simulink model "PosControl_Sim_RPT"  (R2023b)
settings: Solver=ode4  StartTime=0.0  StopTime=3.35  FixedStep=0.001  RelTol=1e-3
InitFcn:
  | Init_control;
values from neighbouring files (symbols this model uses):
  CONSTANTS_ONE_G = 9.8    [Init_control.m]
  DEG2RAD = 0.0174533    [Init_control.m]
  F_xy = [(wn^2+2*sigma*wn*ki)/eps^2, (2*sigma*wn+ki)/eps, ki*wn^2/eps^3, -(wn^2+2*sigma*wn*ki)/eps^2, -(2*sigma*wn+ki)/eps]    [Init_control.m]
  F_z = [(wn^2+2*sigma*wn*ki)/eps^2, (2*sigma*wn+ki)/eps, ki*wn^2/eps^3, -(wn^2+2*sigma*wn*ki)/eps^2, -(2*sigma*wn+ki)/eps]    [Init_control.m]
  FLT_EPSILON = 1e-5    (= 1e-05)    [Init_control.m]
  MAX_CONTROL_ANGLE_RATE_PITCH = 220    [Init_control.m]
  MAX_CONTROL_ANGLE_RATE_ROLL = 220    [Init_control.m]
  MAX_CONTROL_ANGLE_RATE_Y = 200    [Init_control.m]
  MAX_CONTROL_VELOCITY_XY = 5*2    (= 10)    [Init_control.m]
  MAX_CONTROL_VELOCITY_Z = 3*2    (= 6)    [Init_control.m]
  MC_PITCH_P = 6.5    [Init_control.m]
  MC_PITCHRATE_D = 0.0005    [Init_control.m]
  MC_PITCHRATE_I = 0.2    [Init_control.m]
  MC_PITCHRATE_P = 0.06    [Init_control.m]
  MC_ROLL_P = 11.5    [Init_control.m]
  MC_ROLLRATE_D = 0.0005    [Init_control.m]
  MC_ROLLRATE_I = 0.2    [Init_control.m]
  MC_ROLLRATE_P = 0.055    [Init_control.m]
  MC_YAW_P = 2.8    [Init_control.m]
  MC_YAW_WEIGHT = 0.4    [Init_control.m]
  MC_YAWRATE_D = 0.00    (= 0)    [Init_control.m]
  MC_YAWRATE_I = 0.1    [Init_control.m]
  MC_YAWRATE_P = 0.2    [Init_control.m]
  MPC_THR_MAX = 0.9    [Init_control.m]
  MPC_THR_MIN = 0.06    [Init_control.m]
  MPC_THR_XY_MARG = 0.3    [Init_control.m]
  MPC_TILTMAX_AIR = 90    [Init_control.m]
  Saturation_I_az = 5    [Init_control.m]
  Saturation_I_RP_Max = 0.3    [Init_control.m]
  Saturation_I_RP_Min = -0.3    [Init_control.m]
  Saturation_I_Y_Max = 0.2    [Init_control.m]
  Saturation_I_Y_Min = -0.2    [Init_control.m]
  THR_HOVER = 0.331    [Init_control.m]
undefined symbols (not defined in the file or in its folder): DiscIntNeverNeededParam, earthRadius, ModelInit_AngEuler, ModelInit_PosE, ModelInit_Rads, ModelInit_RateB, ModelInit_VelB, ModelParam_envGravityAcc, ModelParam_motorCp, ModelParam_motorCr, ModelParam_motorJm, ModelParam_motorT, ModelParam_motorWb, ModelParam_rotorCm, ModelParam_rotorCt, ModelParam_uavCCm, ModelParam_uavCd, ModelParam_uavJ, ModelParam_uavMass, ModelParam_uavR
libraries: simulink x4, sharedutil x2, aerolibfltsims x2, aerolibanimutils x1
(part 2 of 2)

== matlab function PosControl_Sim_RPT/Control System/Control System/position_control/MATLAB Function1 ==
  data: accx_sp input; thr_sp output; accy_sp input; accz_sp input; CONSTANTS_ONE_G input; DEG2RAD input; MPC_TILTMAX_AIR input; THR_HOVER input; MPC_THR_MIN input; FLT_EPSILON input
function thr_sp = accelerationControl(accx_sp, accy_sp, accz_sp, CONSTANTS_ONE_G, DEG2RAD, MPC_TILTMAX_AIR, THR_HOVER, MPC_THR_MIN, FLT_EPSILON)

selMethod = 2;

if selMethod == 1 % this original method implmented in PX4

    lim_thr_min = MPC_THR_MIN; 

    acc_sp = [accx_sp, accy_sp, accz_sp]';
    thr_sp = zeros(3,1);

    % Assume standard acceleration due to gravity in vertical direction for attitude generation
    body_z = [-acc_sp(1), -acc_sp(2), CONSTANTS_ONE_G]';
    body_z = body_z / norm(body_z);

    lim_tilt = MPC_TILTMAX_AIR * DEG2RAD; 
    limitTilt(body_z, [0, 0, 1]', lim_tilt, FLT_EPSILON);

    % Scale thrust assuming hover thrust produces standard gravity
    hover_thrust = THR_HOVER; 
    collective_thrust = acc_sp(3) * (hover_thrust / CONSTANTS_ONE_G) - hover_thrust;

    % Project thrust to planned body attitude
    collective_thrust = collective_thrust / dot( [0, 0, 1]', body_z );

    collective_thrust = min(collective_thrust, -lim_thr_min);
    thr_sp = body_z * collective_thrust;

else
    lim_thr_min = MPC_THR_MIN; 

    acc_sp = [accx_sp, accy_sp, accz_sp]';
    thr_sp = zeros(3,1);

    % Assume standard acceleration due to gravity in vertical direction for attitude generation
    % body_z = [-acc_sp(1), -acc_sp(2), CONSTANTS_ONE_G]';
    if acc_sp(3) < CONSTANTS_ONE_G 
        body_z = [-acc_sp(1), -acc_sp(2), -acc_sp(3) + CONSTANTS_ONE_G]';
    else
        body_z = [-acc_sp(1), -acc_sp(2), 0]'; % Prevent the drone from flipping upside down
        acc_sp(3) = CONSTANTS_ONE_G; % ma
    end
    body_z = body_z / norm(body_z);

    lim_tilt = MPC_TILTMAX_AIR * DEG2RAD; 
    limitTilt(body_z, [0, 0, 1]', lim_tilt, FLT_EPSILON);

    % Scale thrust assuming hover thrust produces standard gravity
    hover_thrust = THR_HOVER; 
    % collective_thrust = acc_sp(3) * (hover_thrust / CONSTANTS_ONE_G) - hover_thrust;
    
    collective_thrust = - norm(acc_sp + [0, 0, -CONSTANTS_ONE_G]') * (hover_thrust / CONSTANTS_ONE_G); 

    % Project thrust to planned body attitude
%     if dot( [0, 0, 1]', body_z ) > FLT_EPSILON
%         collective_thrust = collective_thrust / dot( [0, 0, 1]', body_z );
%     else
%         collective_thrust = norm(acc_sp) * (hover_thrust / CONSTANTS_ONE_G) - hover_thrust;
%     end

    collective_thrust = min(collective_thrust, -lim_thr_min);
    thr_sp = body_z * collective_thrust;
end 

end


function body_unit = limitTilt(body_unit, world_unit, max_angle, FLT_EPSILON )
    
    % determine tilt
	dot_product_unit = dot(body_unit, world_unit);
	angle = acos(dot_product_unit);
	
    % limit tilt
	angle = min(angle, max_angle);
	rejection = body_unit - (dot_product_unit * world_unit);

	% corner case exactly parallel vectors
	if  norm(rejection)^2 < FLT_EPSILON  
		rejection(1) = 1.0;
    end

	body_unit = cos(angle) * world_unit + sin(angle) * ( rejection/norm(rejection) );

end


% void limitTilt(Vector3f &body_unit, const Vector3f &world_unit, const float max_angle)
% {
% 	// determine tilt
% 	const float dot_product_unit = body_unit.dot(world_unit);
% 	float angle = acosf(dot_product_unit);
% 	// limit tilt
% 	angle = math::min(angle, max_angle);
% 	Vector3f rejection = body_unit - (dot_product_unit * world_unit);
% 
% 	// corner case exactly parallel vectors
% 	if (rejection.norm_squared() < FLT_EPSILON) {
% 		rejection(0) = 1.f;
% 	}
% 
% 	body_unit = cosf(angle) * world_unit + sinf(angle) * rejection.unit();
% }



% // Assume standard acceleration due to gravity in vertical direction for attitude generation
% 	Vector3f body_z = Vector3f(-_acc_sp(0), -_acc_sp(1), CONSTANTS_ONE_G).normalized();
% 	ControlMath::limitTilt(body_z, Vector3f(0, 0, 1), _lim_tilt);
% 	// Scale thrust assuming hover thrust produces standard gravity
% 	float collective_thrust = _acc_sp(2) * (_hover_thrust / CONSTANTS_ONE_G) - _hover_thrust;
% 	// Project thrust to planned body attitude
% 	collective_thrust /= (Vector3f(0, 0, 1).dot(body_z));
% 	collective_thrust = math::min(collective_thrust, -_lim_thr_min);
% 	_thr_sp = body_z * collective_thrust;

== matlab function PosControl_Sim_RPT/Quadcopter Dynamics/Control Effectiveness Model/Propeller Model ==
  data: w input; R input; Fb output; Fd output; Mb output; Cm input; Ct input; Vb input; Cd input; wb input; Md output; Cdm input; Jrp input; Ga output
function [Fb, Fd, Mb, Md, Ga] = fcn(w, R, Cm, Ct, Vb, Cd,wb, Cdm, Jrp)
 %Function description:
 %  Obtain the force and torque acting on the body. The airframe of the
 %  quadrotor is as follows:
 %3↓   1↑
 %  \ /
 %  / \
 %2↑   4↓
 %↑ stands for counterclockwise and ↓stands for clockwise.
 %Input：
 %  w: motor speed，unit：rad/s
 %  R: body radius(m)
 %  Cm: torque coefficient
 %  Ct: thrust coefficient
 %  Vb: aircraft speed in the body coordinate system
 %  Cd: damping coefficient
 %  wb: angular velocity in the body coordinate system
 %  Cdm: damping moment coefficient vector
 %  Jrp:  moment of inertia of motor rotor + propeller
 %Output:
 %  Fb: thrust under the body coordinate system
 %  Fd: aerodynamic force under the body coordinate system
 %  Mb: torque under the body coordinate system
 %  Md: aerodynamic moment
 %  Ga: gyro moment
 M_rctcm = [-sin(pi/4)*R*Ct, sin(pi/4)*R*Ct, sin(pi/4)*R*Ct, -sin(pi/4)*R*Ct;
            sin(pi/4)*R*Ct, -sin(pi/4)*R*Ct, sin(pi/4)*R*Ct, -sin(pi/4)*R*Ct;
            Cm, Cm, -Cm, -Cm];
 Mb = M_rctcm*(w.^2);  % torque
 
 Fb = [0; 0; -sum(Ct*(w.^2))];  % thrust
 Fd = -Cd*Vb.*abs(Vb)*0.5;  % aerodynamic force
 Md = -Cdm.*wb.*abs(wb);  % aerodynamic moment
 % gyro moment
 Ga = zeros(3,1);
 Ga(1) = Jrp*wb(2)*( w(1) + w(2) - w(3) - w(4));
 Ga(2) = Jrp*wb(1)*(-w(1) - w(2) + w(3) + w(4));
end

== matlab function PosControl_Sim_RPT/Control System/Control System/position_control/MATLAB Function2 ==
  data: thr_sp input; q_sp output; yaw_sp input; att_sp output; net_thrust output; FLT_EPSILON input; debug_step_signal input
function [q_sp, att_sp, net_thrust] = thrustToAttitude(thr_sp, yaw_sp, FLT_EPSILON, debug_step_signal)

body_z = -thr_sp;

% zero vector, no direction, set safe level value
if ( sqrt( norm(body_z) ) < FLT_EPSILON ) 
	body_z(3) = 1.0;
end

body_z = body_z / norm(body_z);

% vector of desired yaw direction in XY plane, rotated by PI/2
y_C = [-sin(yaw_sp), cos(yaw_sp), 0.0]';

% desired body_x axis, orthogonal to body_z
body_x = cross(y_C, body_z);

% keep nose to front while inverted upside down
if body_z(3) < 0.0
	body_x = -body_x;
end

if (abs(body_z(3)) < 0.000001) 
	% desired thrust is in XY plane, set X downside to construct correct matrix,
	% but yaw component will not be used actually
	body_x = zeros(3,1);
	body_x(3) = 1.0;
end

body_x = body_x / norm(body_x);

% desired body_y axis
body_y = cross(body_z, body_x);


% fill rotation matrix
R_sp = [body_x, body_y, body_z];

% copy quaternion setpoint to attitude setpoint topic
q_sp = rotm2quat(R_sp);

% calculate euler angles, for logging only, must not be used for control
eul_sp = rotm2eul( R_sp, 'ZYX' );
att_sp = [eul_sp(3), eul_sp(2), eul_sp(1)]';

%*****   for debug only  ********
% if debug_step_signal > 0.5
%     eul_sp = [0, 10*pi/180, 15*pi/180];
% else
%     eul_sp = [0, 0*pi/180, 0*pi/180];
% end
% att_sp = [eul_sp(3), eul_sp(2), eul_sp(1)]';
% R_sp = eul2rotm( eul_sp);
% q_sp = rotm2quat(R_sp);
%******** end of debug code *******

% the thrust on body axis
thrust_body = -norm(thr_sp);

net_thrust = - thrust_body; % designed thrust generated by motors, which is non-negative 
end





% // zero vector, no direction, set safe level value
% 	if (body_z.norm_squared() < FLT_EPSILON) {
% 		body_z(2) = 1.f;
% 	}
% 
% 	body_z.normalize();
% 
% 	// vector of desired yaw direction in XY plane, rotated by PI/2
% 	const Vector3f y_C{-sinf(yaw_sp), cosf(yaw_sp), 0.f};
% 
% 	// desired body_x axis, orthogonal to body_z
% 	Vector3f body_x = y_C % body_z;
% 
% 	// keep nose to front while inverted upside down
% 	if (body_z(2) < 0.0f) {
% 		body_x = -body_x;
% 	}
% 
% 	if (fabsf(body_z(2)) < 0.000001f) {
% 		// desired thrust is in XY plane, set X downside to construct correct matrix,
% 		// but yaw component will not be used actually
% 		body_x.zero();
% 		body_x(2) = 1.0f;
% 	}
% 
% 	body_x.normalize();
% 
% 	// desired body_y axis
% 	const Vector3f body_y = body_z % body_x;
% 
% 	Dcmf R_sp;
% 
% 	// fill rotation matrix
% 	for (int i = 0; i < 3; i++) {
% 		R_sp(i, 0) = body_x(i);
% 		R_sp(i, 1) = body_y(i);
% 		R_sp(i, 2) = body_z(i);
% 	}
% 
% 	// copy quaternion setpoint to attitude setpoint topic
% 	const Quatf q_sp{R_sp};
% 	q_sp.copyTo(att_sp.q_d);
% 
% 	// calculate euler angles, for logging only, must not be used for control
% 	const Eulerf euler{R_sp};
% 	att_sp.roll_body = euler.phi();
% 	att_sp.pitch_body = euler.theta();
% 	att_sp.yaw_body = euler.psi();

== matlab function PosControl_Sim_RPT/Control System/Control System/MATLAB Function ==
  data: trigger input; q_sp output
function q_sp  = q_sp_debug(trigger)

if trigger > 0.5
    eul_sp = [0*pi/180, 30*pi/180, 0*pi/180]; % 'ZYX': eul_sp = [yaw_sp, roll_sep, pitch_sp]
else
    eul_sp = [0, 0*pi/180, 0*pi/180];
end
att_sp = [eul_sp(3), eul_sp(2), eul_sp(1)]';
R_sp = eul2rotm( eul_sp);
q_sp = rotm2quat(R_sp);

== matlab function PosControl_Sim_RPT/Quadcopter Dynamics/Propulsor Model/Throttle To rads Gain _1/PWM to RPM ==
  data: u input; y output; Cp input
function y = fcn(u, Cp)

y = Cp(1) * u^2 + Cp(2) * u + Cp(3);

== matlab function PosControl_Sim_RPT/Quadcopter Dynamics/Propulsor Model/Throttle To rads Gain _2/PWM to RPM ==
  data: u input; y output; Cp input
function y = fcn(u, Cp)

y = Cp(1) * u^2 + Cp(2) * u + Cp(3);

== matlab function PosControl_Sim_RPT/Quadcopter Dynamics/Propulsor Model/Throttle To rads Gain _3/PWM to RPM ==
  data: u input; y output; Cp input
function y = fcn(u, Cp)

y = Cp(1) * u^2 + Cp(2) * u + Cp(3);

== matlab function PosControl_Sim_RPT/Quadcopter Dynamics/Propulsor Model/Throttle To rads Gain _4/PWM to RPM ==
  data: u input; y output; Cp input
function y = fcn(u, Cp)

y = Cp(1) * u^2 + Cp(2) * u + Cp(3);

== matlab function PosControl_Sim_RPT/Control System/InputConditioning/deadzone1 ==
  data: u input; y output
function y = fcn(u)
%Function description:
%  Control the range of the remote control input from RCMin to RCMax, and
%  set a dead zone with a dead zone size of ±deadZone. The output y is
%  normalized to 0~1.You can get the RC calibration parameters in QGC.
RCMin = 1100;
RCMax = 1900;
RCMid = (RCMin + RCMax)/2;
deadZoneRate = 0.05;
deadZone = deadZoneRate*(RCMax - RCMin);
k = 1/(RCMax - RCMid - deadZone);
% saturation
if(u < RCMin)
    u = RCMin;
elseif(u > RCMax)
    u = RCMax;
end
% dead zone and normalize
 if(u > RCMid + deadZone)
    y = (u-RCMid - deadZone)*k;
 elseif(u < RCMid - deadZone)
     y = (u - RCMid + deadZone)*k;
 else
     y = 0;
 end

 end

== matlab function PosControl_Sim_RPT/Control System/InputConditioning/deadzone2 ==
  data: u input; y output
function y = fcn(u)
%Function description:
%  Control the range of the remote control input from RCMin to RCMax, and
%  set a dead zone with a dead zone size of ±deadZone. The output y is
%  normalized to 0~1.You can get the RC calibration parameters in QGC.
RCMin = 1100;
RCMax = 1900;
RCMid = (RCMin + RCMax)/2;
deadZoneRate = 0.05;
deadZone = deadZoneRate*(RCMax - RCMin);
k = 1/(RCMax - RCMid - deadZone);
% saturation
if(u < RCMin)
    u = RCMin;
elseif(u > RCMax)
    u = RCMax;
end
% dead zone and normalize
 if(u > RCMid + deadZone)
    y = (u-RCMid - deadZone)*k;
 elseif(u < RCMid - deadZone)
     y = (u - RCMid + deadZone)*k;
 else
     y = 0;
 end

 end

== matlab function PosControl_Sim_RPT/Control System/InputConditioning/deadzone3 ==
  data: u input; y output
function y = fcn(u)
%Function description:
%  Control the range of the remote control input from RCMin to RCMax, and
%  set a dead zone with a dead zone size of ±deadZone. The output y is
%  normalized to 0~1.You can get the RC calibration parameters in QGC.
RCMin = 1100;
RCMax = 1900;
RCMid = (RCMin + RCMax)/2;
deadZoneRate = 0.05;
deadZone = deadZoneRate*(RCMax - RCMin);
k = 1/(RCMax - RCMid - deadZone);
% saturation
if(u < RCMin)
    u = RCMin;
elseif(u > RCMax)
    u = RCMax;
end
% dead zone and normalize
 if(u > RCMid + deadZone)
    y = (u-RCMid - deadZone)*k;
 elseif(u < RCMid - deadZone)
     y = (u - RCMid + deadZone)*k;
 else
     y = 0;
 end

 end

== matlab function PosControl_Sim_RPT/Control System/InputConditioning/deadzone4 ==
  data: u input; y output
function y = fcn(u)
%Function description:
%  Control the range of the remote control input from RCMin to RCMax, and
%  set a dead zone with a dead zone size of ±deadZone. The output y is
%  normalized to 0~1.You can get the RC calibration parameters in QGC.
RCMin = 1100;
RCMax = 1900;
RCMid = (RCMin + RCMax)/2;
deadZoneRate = 0.05;
deadZone = deadZoneRate*(RCMax - RCMin);
k = 1/(RCMax - RCMid - deadZone);
% saturation
if(u < RCMin)
    u = RCMin;
elseif(u > RCMax)
    u = RCMax;
end
% dead zone and normalize
 if(u > RCMid + deadZone)
    y = (u-RCMid - deadZone)*k;
 elseif(u < RCMid - deadZone)
     y = (u - RCMid + deadZone)*k;
 else
     y = 0;
 end

 end

== matlab function PosControl_Sim_RPT/Control System/Control System/pwm_out1 ==
  data: Roll input; M1 output; Pitch input; Yaw input; Thrust input; M2 output; M3 output; M4 output
function [M1, M2, M3, M4] = motor_mixer(Roll, Pitch, Yaw, Thrust)
%Function description:
%  Control allocation. The quadrotor type is X-configuration,
%  and the airframe is as follows:
%3↓   1↑
 %  \ /
 %  / \
 %2↑   4↓
%Input：
%  Roll, Pitch, Yaw: attitude controller output.
%  Thrust

idle_PWM = 1000;
scale = 1000;

M1 = (Thrust - Roll + Pitch + Yaw) * scale + idle_PWM;
M2 = (Thrust + Roll - Pitch + Yaw) * scale + idle_PWM;
M3 = (Thrust + Roll + Pitch - Yaw) * scale + idle_PWM;
M4 = (Thrust - Roll - Pitch - Yaw) * scale + idle_PWM;

== matlab function PosControl_Sim_RPT/Control System/Control System/AttitudeControl/MATLAB Function ==
  data: att_q input; att_setpoint_q input; rate_setpoint output; qd output; yawrate_d input; Kp_ROLL_ANGLE input; Kp_PITCH_ANGLE input; Kp_YAW_ANGLE input; MC_YAW_WEIGHT input; qd2 output
function [rate_setpoint, qd, qd2]  = AttitudeControl(att_q, att_setpoint_q, yawrate_d, Kp_ROLL_ANGLE, Kp_PITCH_ANGLE, Kp_YAW_ANGLE, MC_YAW_WEIGHT)

%******* for debug *****
% qd_red = zeros(1,4);
% q_mix = zeros(1,4);
%******* end of debug *****

q  = [att_q(1), att_q(2), att_q(3), att_q(4)];
qd = [att_setpoint_q(1), att_setpoint_q(2), att_setpoint_q(3), att_setpoint_q(4)];
% qd2 = qd; % for debug only
    
% calcuate reduced desired attitude neglecting vehicle's yaw to
% prioritize roll and pitch
rotm = quat2rotm(q); 
e_z = rotm(:,3);
rotm_d = quat2rotm(qd);
e_z_d = rotm_d(:,3);
    
% n = zeros(3,1);
% n = cross(e_z, e_z_d)/norm(cross(e_z, e_z_d));
% a = atan2( cross(e_z, e_z_d), dot(e_z, e_z_d) );
%     
% qd_red = [ cos(a/2), sin(a/2) *n(1), sin(a/2) *n(2), sin(a/2) *n(3)];

qd_red = Quat2Vec(e_z, e_z_d); 

if ( abs(qd_red(2)) > (1.0 - 1e-5) ) || ( abs(qd_red(3)) > (1.0 - 1e-5) ) 
    % In the infinitesimal corner case where the vehicle and thrust have the completely opposite direction,
    % full attitude control anyways generates no yaw input and directly takes the combination of
	% roll and pitch leading to the correct desired yaw. Ignoring this case would still be totally safe and stable.
	qd_red = qd;

else
    % transform rotation from current to desired thrust vector into a world frame reduced desired attitude
	qd_red = quatmultiply( qd_red, q );
end

qd2 = qd_red; % for debug only 

% mix full and reduced desired attitude
q_mix = quatmultiply( quatinv(qd_red), qd);
% q_mix.canonicalize();
if abs( q_mix(1) ) > 1E-5
    q_mix = q_mix * sign(q_mix(1)); 
end
    

% catch numerical problems with the domain of acosf and asinf
q_mix(1) = min( max(q_mix(1), -1.0), 1.0);
q_mix(4) = min( max(q_mix(4), -1.0), 1.0);
yaw_w = MC_YAW_WEIGHT; 

qd_ = quatmultiply( qd_red, [cos(yaw_w * acos(q_mix(1))), 0, 0, sin(yaw_w * asin(q_mix(4))) ]  );
qd = qd_(1,:); 

% quaternion attitude control law, qe is rotation from q to qd
qe = quatmultiply(quatinv(q), qd);

    
% using sin(alpha/2) scaled rotation axis as attitude error (see quaternion definition by axis angle)
% also taking care of the antipodal unit quaternion ambiguity
% canonicalize();
if abs( qe(1) ) > 1E-5
    qe = qe * sign(qe(1)); 
end 
eq = 2.0 * [qe(2), qe(3), qe(4)];

% calculate angular rates setpoint
Kp_roll  = Kp_ROLL_ANGLE;
Kp_pitch = Kp_PITCH_ANGLE;
Kp_yaw   = Kp_YAW_ANGLE; 

rate_setpoint = zeros(3,1); 
rate_setpoint = [Kp_roll*eq(1), Kp_pitch*eq(2), Kp_yaw*eq(3)]';

% Feed forward the yaw setpoint rate.
% yawspeed_setpoint is the feed forward commanded rotation around the world z-axis,
% but we need to apply it in the body frame (because _rates_sp is expressed in the body frame).
% Therefore we infer the world z-axis (expressed in the body frame) by taking the last column of R.transposed (== q.inversed)
% and multiply it by the yaw setpoint rate (yawspeed_setpoint).
% This yields a vector representing the commanded rotatation around the world z-axis expressed in the body frame
% such that it can be added to the rates setpoint.

if( isfinite(yawrate_d) )
    rotm_t = quat2rotm( quatinv(q) ); 
    rate_setpoint = rate_setpoint + rotm_t(:,3) * yawrate_d; 
end

% limit rates 
% rate_limit = zero(3);
% rate_limit(1) = MAX_CONTROL_ANGLE_RATE_ROLL; 
% rate_limit(2) = MAX_CONTROL_ANGLE_RATE_PITCH; 
% rate_limit(3) = MAX_CONTROL_ANGLE_RATE_YAW; 
% 
% for i=1:3
%     rate_setpoint(i) = min( max(q_mix(1), -rate_limit(i)), rate_limit(i));
% end


end


%%
% Quaternion from two vectors
% Generates shortest rotation from source to destination vector
%
% @param dst destination vector (no need to normalize)
% @param src source vector (no need to normalize)
% @param eps epsilon threshold which decides if a value is considered zero

function	q = Quat2Vec( src, dst )

q = zeros(1,4); 

eps = 1e-5; 
cr = cross(src, dst);
dt = dot(src, dst);

if (norm(cr) < eps && dt < 0) 
% handle corner cases with 180 degree rotations
% if the two vectors are parallel, cross product is zero
% if they point opposite, the dot product is negative

    cr = abs(src);

    if (cr(1) < cr(2)) 
        if (cr(1) < cr(3)) 
            cr = [1, 0, 0]';
        else 
            cr = [0, 0, 1]';
        end
     else 
        if (cr(2) < cr(3)) 
            cr = [0, 1, 0]';
        else 
            cr = [0, 0, 1]';
        end
    end

	q(1) = 0;
	cr = cross(src, cr);

else 
	% normal case, do half-way quaternion solution
	q(1) = dt + sqrt( (norm(src))^2 * (norm(dst))^2 );
end

	q(2) = cr(1);
	q(3) = cr(2);
	q(4) = cr(3);
	q = quatnormalize(q);
end








% /**
% 	 * Quaternion from two vectors
% 	 * Generates shortest rotation from source to destination vector
% 	 *
% 	 * @param dst destination vector (no need to normalize)
% 	 * @param src source vector (no need to normalize)
% 	 * @param eps epsilon threshold which decides if a value is considered zero
% 	 */
% 	Quaternion(const Vector3<Type> &src, const Vector3<Type> &dst, const Type eps = Type(1e-5))
% 	{
% 		Quaternion &q = *this;
% 		Vector3<Type> cr = src.cross(dst);
% 		const float dt = src.dot(dst);
% 
% 		if (cr.norm() < eps && dt < 0) {
% 			// handle corner cases with 180 degree rotations
% 			// if the two vectors are parallel, cross product is zero
% 			// if they point opposite, the dot product is negative
% 			cr = src.abs();
% 
% 			if (cr(0) < cr(1)) {
% 				if (cr(0) < cr(2)) {
% 					cr = Vector3<Type>(1, 0, 0);
% 
% 				} else {
% 					cr = Vector3<Type>(0, 0, 1);
% 				}
% 
% 			} else {
% 				if (cr(1) < cr(2)) {
% 					cr = Vector3<Type>(0, 1, 0);
% 
% 				} else {
% 					cr = Vector3<Type>(0, 0, 1);
% 				}
% 			}
% 
% 			q(0) = Type(0);
% 			cr = src.cross(cr);
% 
% 		} else {
% 			// normal case, do half-way quaternion solution
% 			q(0) = dt + std::sqrt(src.norm_squared() * dst.norm_squared());
% 		}
% 
% 		q(1) = cr(0);
% 		q(2) = cr(1);
% 		q(3) = cr(2);
% 		q.normalize();
% 	}


    
    
%%--------------------------------------------------------------------    
    
% matrix::Vector3f AttitudeControl::update(const Quatf &q) const
% {    
%   Quatf qd = _attitude_setpoint_q;
% 
% 	// calculate reduced desired attitude neglecting vehicle's yaw to prioritize roll and pitch
% 	const Vector3f e_z = q.dcm_z();
% 	const Vector3f e_z_d = qd.dcm_z();
% 	Quatf qd_red(e_z, e_z_d);
% 
% 	if (fabsf(qd_red(1)) > (1.f - 1e-5f) || fabsf(qd_red(2)) > (1.f - 1e-5f)) {
% 		// In the infinitesimal corner case where the vehicle and thrust have the completely opposite direction,
% 		// full attitude control anyways generates no yaw input and directly takes the combination of
% 		// roll and pitch leading to the correct desired yaw. Ignoring this case would still be totally safe and stable.
% 		qd_red = qd;
% 
% 	} else {
% 		// transform rotation from current to desired thrust vector into a world frame reduced desired attitude
% 		qd_red *= q;
% 	}
% 
% 	// mix full and reduced desired attitude
% 	Quatf q_mix = qd_red.inversed() * qd;
% 	q_mix.canonicalize();
% 	// catch numerical problems with the domain of acosf and asinf
% 	q_mix(0) = math::constrain(q_mix(0), -1.f, 1.f);
% 	q_mix(3) = math::constrain(q_mix(3), -1.f, 1.f);
% 	qd = qd_red * Quatf(cosf(_yaw_w * acosf(q_mix(0))), 0, 0, sinf(_yaw_w * asinf(q_mix(3))));
% 
% 	// quaternion attitude control law, qe is rotation from q to qd
% 	const Quatf qe = q.inversed() * qd;
% 
% 	// using sin(alpha/2) scaled rotation axis as attitude error (see quaternion definition by axis angle)
% 	// also taking care of the antipodal unit quaternion ambiguity
% 	const Vector3f eq = 2.f * qe.canonical().imag();
% 
% 	// calculate angular rates setpoint
% 	matrix::Vector3f rate_setpoint = eq.emult(_proportional_gain);
% 
% 	// Feed forward the yaw setpoint rate.
% 	// yawspeed_setpoint is the feed forward commanded rotation around the world z-axis,
% 	// but we need to apply it in the body frame (because _rates_sp is expressed in the body frame).
% 	// Therefore we infer the world z-axis (expressed in the body frame) by taking the last column of R.transposed (== q.inversed)
% 	// and multiply it by the yaw setpoint rate (yawspeed_setpoint).
% 	// This yields a vector representing the commanded rotatation around the world z-axis expressed in the body frame
% 	// such that it can be added to the rates setpoint.
% 	if (std::isfinite(_yawspeed_setpoint)) {
% 		rate_setpoint += q.inversed().dcm_z() * _yawspeed_setpoint;
% 	}
% 
% 	// limit rates
% 	for (int i = 0; i < 3; i++) {
% 		rate_setpoint(i) = math::constrain(rate_setpoint(i), -_rate_limit(i), _rate_limit(i));
% 	}
% 
% 	return rate_setpoint;    
%}

== matlab function PosControl_Sim_RPT/Control System/Control System/position_control/MATLAB Function ==
  data: thr_sp input; thr_sp output; MPC_THR_MAX input; MPC_THR_XY_MARG input
function thr_sp = saturateThrust(thr_sp, MPC_THR_MAX, MPC_THR_XY_MARG)
% This function implements the segment following _accelerationControl() 
% within _velocityControl. Its purpose is to cap or limit the thrust output.

lim_thr_max = MPC_THR_MAX;
lim_thr_xy_margin = MPC_THR_XY_MARG;

% Prioritize vertical control while keeping a horizontal margin
thrust_sp_xy = thr_sp(1:2);
thrust_sp_xy_norm = norm(thrust_sp_xy);
thrust_max_squared = (lim_thr_max)^2;

% Determine how much vertical thrust is left keeping horizontal margin
allocated_horizontal_thrust = min(thrust_sp_xy_norm, lim_thr_xy_margin);
thrust_z_max_squared = thrust_max_squared - (allocated_horizontal_thrust)^2;

% Saturate maximal vertical thrust
thr_sp(3) = max( thr_sp(3), -sqrt(thrust_z_max_squared) );

% Determine how much horizontal thrust is left after prioritizing vertical control
thrust_max_xy_squared = thrust_max_squared - (thr_sp(3))^2;
thrust_max_xy = 0;

if (thrust_max_xy_squared > 0) 
	thrust_max_xy = sqrt(thrust_max_xy_squared);
end

% Saturate thrust in horizontal direction
if (thrust_sp_xy_norm > thrust_max_xy) 
	thr_sp(1:2) = thrust_sp_xy / thrust_sp_xy_norm * thrust_max_xy;
end
    
end
    
    
 

% void PositionControl::_velocityControl(const float dt)
% {
% 	// PID velocity control
% 	Vector3f vel_error = _vel_sp - _vel;
% 	Vector3f acc_sp_velocity = vel_error.emult(_gain_vel_p) + _vel_int - _vel_dot.emult(_gain_vel_d);
% 
% 	// No control input from setpoints or corresponding states which are NAN
% 	ControlMath::addIfNotNanVector3f(_acc_sp, acc_sp_velocity);
% 
% 	_accelerationControl();
% 
% 	// Integrator anti-windup in vertical direction
% 	if ((_thr_sp(2) >= -_lim_thr_min && vel_error(2) >= 0.0f) ||
% 	    (_thr_sp(2) <= -_lim_thr_max && vel_error(2) <= 0.0f)) {
% 		vel_error(2) = 0.f;
% 	}
% 
% 	// Prioritize vertical control while keeping a horizontal margin
% 	const Vector2f thrust_sp_xy(_thr_sp);
% 	const float thrust_sp_xy_norm = thrust_sp_xy.norm();
% 	const float thrust_max_squared = math::sq(_lim_thr_max);
% 
% 	// Determine how much vertical thrust is left keeping horizontal margin
% 	const float allocated_horizontal_thrust = math::min(thrust_sp_xy_norm, _lim_thr_xy_margin);
% 	const float thrust_z_max_squared = thrust_max_squared - math::sq(allocated_horizontal_thrust);
% 
% 	// Saturate maximal vertical thrust
% 	_thr_sp(2) = math::max(_thr_sp(2), -sqrtf(thrust_z_max_squared));
% 
% 	// Determine how much horizontal thrust is left after prioritizing vertical control
% 	const float thrust_max_xy_squared = thrust_max_squared - math::sq(_thr_sp(2));
% 	float thrust_max_xy = 0;
% 
% 	if (thrust_max_xy_squared > 0) {
% 		thrust_max_xy = sqrtf(thrust_max_xy_squared);
% 	}
% 
% 	// Saturate thrust in horizontal direction
% 	if (thrust_sp_xy_norm > thrust_max_xy) {
% 		_thr_sp.xy() = thrust_sp_xy / thrust_sp_xy_norm * thrust_max_xy;
% 	}
% 
% 	// Use tracking Anti-Windup for horizontal direction: during saturation, the integrator is used to unsaturate the output
% 	// see Anti-Reset Windup for PID controllers, L.Rundqwist, 1990
% 	const Vector2f acc_sp_xy_produced = Vector2f(_thr_sp) * (CONSTANTS_ONE_G / _hover_thrust);
% 	const float arw_gain = 2.f / _gain_vel_p(0);
% 
% 	// The produced acceleration can be greater or smaller than the desired acceleration due to the saturations and the actual vertical thrust (computed independently).
% 	// The ARW loop needs to run if the signal is saturated only.
% 	const Vector2f acc_sp_xy = _acc_sp.xy();
% 	const Vector2f acc_limited_xy = (acc_sp_xy.norm_squared() > acc_sp_xy_produced.norm_squared())
% 					? acc_sp_xy_produced
% 					: acc_sp_xy;
% 	vel_error.xy() = Vector2f(vel_error) - arw_gain * (acc_sp_xy - acc_limited_xy);
% 
% 	// Make sure integral doesn't get NAN
% 	ControlMath::setZeroIfNanVector3f(vel_error);
% 	// Update integral part of velocity control
% 	_vel_int += vel_error.emult(_gain_vel_i) * dt;
% 
% 	// limit thrust integral
% 	_vel_int(2) = math::min(fabsf(_vel_int(2)), CONSTANTS_ONE_G) * sign(_vel_int(2));
% }

== matlab function PosControl_Sim_RPT/Quadcopter Dynamics/Rigid Model/Rigid-Body Kinematic Model /Quaternion to rotation matrix ==
  data: q input; Reb output
function Reb = fcn(q)
%Function description;
%  The rotation matrix of the Aircraft-Body Coordinate Frame (ABCF) to the
%  Earth-Fixed Coordinate Frame (EFCF) is obtained from the quaternions
Reb = [q(1)*q(1) + q(2)*q(2) - q(3)*q(3) - q(4)*q(4), 2*(q(2)*q(3) - q(1)*q(4)), 2*(q(2)*q(4) + q(1)*q(3))
           2*(q(2)*q(3) + q(1)*q(4)), q(1)*q(1) - q(2)*q(2) + q(3)*q(3) - q(4)*q(4), 2*(q(3)*q(4) - q(1)*q(2))
           2*(q(2)*q(4) - q(1)*q(3)), 2*(q(3)*q(4) + q(1)*q(2)), q(1)*q(1) - q(2)*q(2) - q(3)*q(3) + q(4)*q(4)];

== matlab function PosControl_Sim_RPT/Quadcopter Dynamics/Rigid Model/Rigid-Body Kinematic Model /Quaternion to Euler ==
  data: q input; y output
function y = fcn(q)
 %Function description:
%  Quaternions to Euler
phi = atan2(2*(q(1)*q(2) + q(3)*q(4)), (1 - 2*(q(2)*q(2) + q(3)*q(3))));
theta = asin(2*(q(1)*q(3) - q(2)*q(4)));
psi = atan2(2*(q(1)*q(4) + q(2)*q(3)), (1 - 2*(q(3)*q(3) + q(4)*q(4))));
y = [phi theta psi];
